simulink model "PM_fnc17_DevHarness_rate_limiter"  (R2022a)
settings: Solver=FixedStepAuto  StartTime=0.0  StopTime=inf  FixedStep=fixedsteprate_s  RelTol=1e-3
values from neighbouring files (symbols this model uses):
  fixedsteprate_s = rate_s    (= 0.01)    [PM_fnc1000_tc01_iter01_testsignal_builder.m]    (also in PM_fnc21_tc01_iter01_testsignal_builder.m; PM_fnc22_tc01_iter01_testsignal_builder.m)
settings Model: Creator=306427  LastModifiedBy=306427

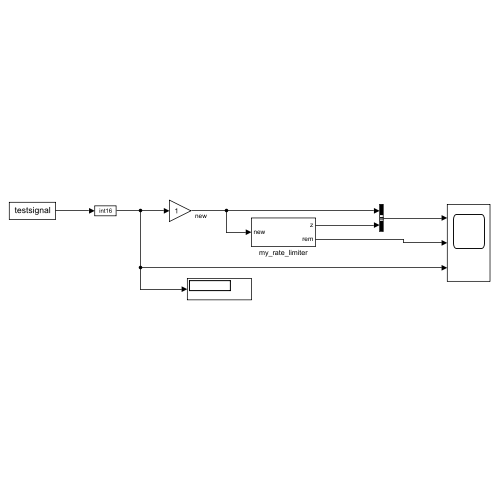
[thumbnail: Simulink's stored preview of the top-level diagram]
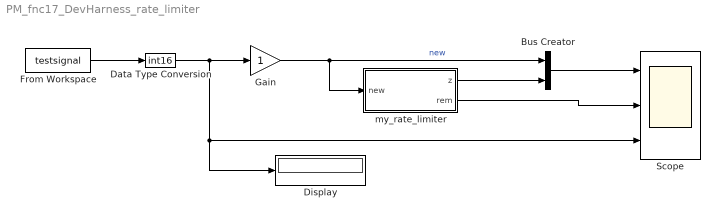
== system PM_fnc17_DevHarness_rate_limiter ==
  Bus Creator : BusCreator  Inputs=2
  Data Type Conversion : DataTypeConversion  OutDataTypeStr=int16  SaturateOnIntegerOverflow=off  RndMeth=Floor
  Display : Display
  From Workspace : FromWorkspace  VariableName=testsignal  SampleTime=fixedsteprate_s
  Gain : Gain  OutDataTypeStr=int16  ParamDataTypeStr=Inherit: Same as input
  Scope : Scope  NumInputPorts=3
  my_rate_limiter : Subsystem
  wires:
  Gain/1 -> my_rate_limiter/1(new), Bus Creator/1  "new"
  Bus Creator/1 -> Scope/1
  my_rate_limiter/1(z) -> Bus Creator/2
  my_rate_limiter/2(rem) -> Scope/2
  From Workspace/1 -> Data Type Conversion/1
  Data Type Conversion/1 -> Scope/3, Display/1, Gain/1

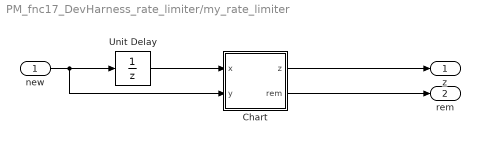
== system PM_fnc17_DevHarness_rate_limiter/my_rate_limiter ==
  new : Inport
  Chart : Stateflow chart  TreatAsAtomicUnit=on
  Unit Delay : UnitDelay  SampleTime=-1  HasFrameUpgradeWarning=on
  z : Outport
  rem : Outport  Port=2
  wires:
  Unit Delay/1 -> Chart/1(x)
  new/1 -> Chart/2(y), Unit Delay/1
  Chart/1(z) -> z/1
  Chart/2(rem) -> rem/1

== stateflow chart PM_fnc17_DevHarness_rate_limiter/my_rate_limiter/Chart ==
  state ZERO_REMAINDER
    prev = x;
    next = y;
    inst_delta = next - prev;
  state NON_ZERO_REMAINDER
    prev = x;
    next = y;
    inst_delta = next - prev;
  (default) -> ZERO_REMAINDER
  ZERO_REMAINDER -> ZERO_REMAINDER [order 2] : [inst_delta <= 10 && inst_delta >= -10]/{...
      | z = next;}
  ZERO_REMAINDER -> NON_ZERO_REMAINDER [order 1] : [inst_delta > 10]/{...
      | z = prev + 10; prev_step = z;
      | remainder = inst_delta - 10;
      | rem = remainder;}
  ZERO_REMAINDER -> NON_ZERO_REMAINDER [order 3] : [inst_delta < -10]/{ ...
      | z = prev - 10; prev_step = z;
      | remainder = inst_delta + 10;
      | rem = remainder;}
  NON_ZERO_REMAINDER -> ZERO_REMAINDER [order 1] : [remainder == 0]
  NON_ZERO_REMAINDER -> NON_ZERO_REMAINDER [order 3] : [inst_delta <= 10 && inst_delta >= -10 && remainder < 0]/{...
      | z = prev_step - 10; prev_step = z;
      | remainder = remainder + 10;
      | rem = remainder;}
  NON_ZERO_REMAINDER -> NON_ZERO_REMAINDER [order 2] : [inst_delta <= 10 && inst_delta >= -10 && remainder > 0]/{...
      | z = prev_step + 10; prev_step = z;
      | remainder = remainder - 10;
      | rem = remainder;}
  data: x input; prev local int16; y input; z output int16; next local int16; remainder local int16; inst_delta local int16; prev_step local int16; rem output int16
